simulink library "rot_grc"  (R2024a)
settings: Solver=VariableStepAuto  StartTime=0.0  StopTime=10.0  RelTol=1e-3
undefined symbols (not defined in the file or in its folder): AROT_ParkCompAngle_X_rpm, ENUM_SENSORFOCMODE_RDCALIGN, KFOC_PolePairs_p, KROT_agOffset_C, KROT_bUseVariableFc_flg, KROT_CurLoopPrd_t, KROT_RotAngleE_rad_ovrdflg, KROT_RotAngleE_rad_ovrdval, KROT_RotSpdMRaw_rpm_ovrdflg, KROT_RotSpdMRaw_rpm_ovrdval, KROT_SpdCutoffFreq_Hz, MROT_ParkCompAngle_Y_rad, MROT_VolPosnOffsWiSpd_Y_deg, ZERO_FLOAT
libraries: GRC_Lib x1
settings Model: Creator=FVT22063  LastModifiedBy=FVT22063

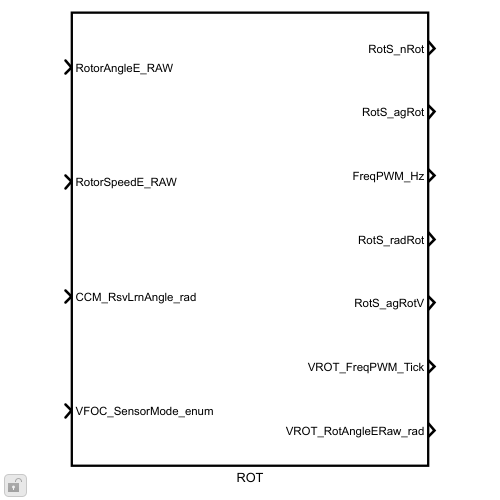
[thumbnail: Simulink's stored preview of the top-level diagram]
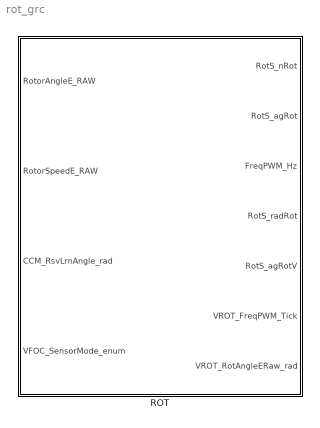
== system rot_grc ==
  ROT : Subsystem  TreatAsAtomicUnit=on

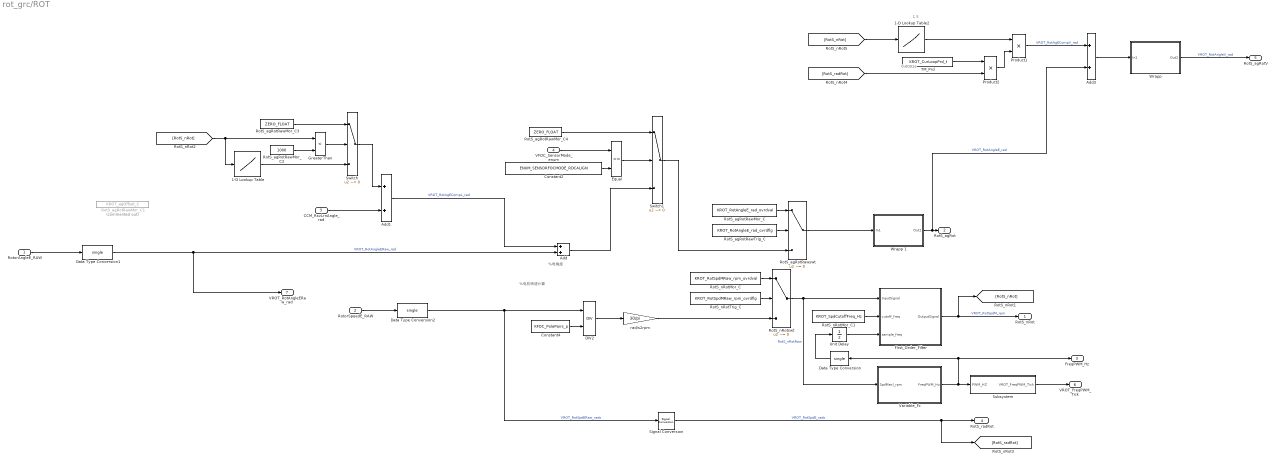
== system rot_grc/ROT ==
  note: 1.5
  note: 0.0001s
  note: %电机转速计算
  note: %电角度
  RotorAngleE_RAW : Inport
  RotorSpeedE_RAW : Inport  Port=2
  CCM_RsvLrnAngle_rad : Inport  Port=3  OutDataTypeStr=single
  VFOC_SensorMode_enum : Inport  Port=4
  1-D Lookup Table : Lookup_n-D  NumberOfTableDimensions=1  BreakpointsForDimension1=AROT_ParkCompAngle_X_rpm  Table=MROT_ParkCompAngle_Y_rad  ExtrapMethod=Clip  UseLastTableValue=on  InternalRulePriority=Speed  RndMeth=Simplest
  1-D Lookup Table2 : Lookup_n-D  NumberOfTableDimensions=1  BreakpointsForDimension1=AROT_ParkCompAngle_X_rpm  Table=MROT_VolPosnOffsWiSpd_Y_deg  ExtrapMethod=Clip  UseLastTableValue=on  InternalRulePriority=Speed  RndMeth=Simplest
  Add : Sum
  Add1 : Sum
  Add3 : Sum
  Constant2 : Constant  Value=ENUM_SENSORFOCMODE_RDCALIGN
  Constant4 : Constant  Value=KFOC_PolePairs_p
  DIV2 : GRC_Lib/ArithmeticOperations/DIV  MinDivVal=1e-15  IpDT=single
  Data Type Conversion : DataTypeConversion  OutDataTypeStr=single  SaturateOnIntegerOverflow=off  RndMeth=Floor
  Data Type Conversion1 : DataTypeConversion  OutDataTypeStr=single  SaturateOnIntegerOverflow=off  RndMeth=Floor
  Data Type Conversion2 : DataTypeConversion  OutDataTypeStr=single  SaturateOnIntegerOverflow=off  RndMeth=Floor
  Equal : RelationalOperator  Operator===  OutDataTypeStr=boolean  RndMeth=Simplest  InputSameDT=off
  First_Order_Filter : Subsystem  AncestorBlock=Library/First_Order_Filter  TreatAsAtomicUnit=on  RTWFcnName=First_Order_Filter
      settings: RTWFcnNameOpts=User specified
  GreaterThan : RelationalOperator  Operator=<  OutDataTypeStr=boolean  RndMeth=Simplest  InputSameDT=off
  Product1 : Product  RndMeth=Zero
  Product2 : Product  RndMeth=Zero
  RotS_agRotRawMor_C : Constant  Value=KROT_RotAngleE_rad_ovrdval
  RotS_agRotRawMor_C1 : Constant  Commented=on  Value=KROT_agOffset_C
  RotS_agRotRawMor_C2 : Constant  Value=1000
  RotS_agRotRawMor_C3 : Constant  Value=ZERO_FLOAT
  RotS_agRotRawMor_C4 : Constant  Value=ZERO_FLOAT
  RotS_agRotRawTrig_C : Constant  Value=KROT_RotAngleE_rad_ovrdflg
  RotS_agRotRawswt : Switch  Criteria=u2 ~= 0  SaturateOnIntegerOverflow=off  InputSameDT=off
  RotS_nRotMor_C : Constant  Value=KROT_RotSpdMRaw_rpm_ovrdval
  RotS_nRotMor_C1 : Constant  Value=KROT_SpdCutoffFreq_Hz  OutDataTypeStr=single
  RotS_nRotTrig_C : Constant  Value=KROT_RotSpdMRaw_rpm_ovrdflg
  RotS_nRotswt : Switch  Criteria=u2 ~= 0  SaturateOnIntegerOverflow=off  InputSameDT=off
  Signal Conversion : SignalConversion  OverrideOpt=off
  Subsystem : Subsystem
  Switch : Switch  Criteria=u2 ~= 0  SaturateOnIntegerOverflow=off  InputSameDT=off
  Switch1 : Switch  Criteria=u2 ~= 0  SaturateOnIntegerOverflow=off  InputSameDT=off
  TM_Prd : Constant  Value=KROT_CurLoopPrd_t  OutDataTypeStr=single
  Unit Delay : UnitDelay  InitialCondition=5000  SampleTime=-1  HasFrameUpgradeWarning=on
  Variable_Fc : Subsystem
  "Wrapp " : Subsystem
  Wrapp 1 : Subsystem
  rad/s2rpm : Gain  Gain=30/pi
  RotS_nRot : Outport  OutDataTypeStr=single  VectorParamsAs1DForOutWhenUnconnected=off
  RotS_agRot : Outport  Port=2  OutDataTypeStr=single  VectorParamsAs1DForOutWhenUnconnected=off
  FreqPWM_Hz : Outport  Port=3  OutDataTypeStr=uint16  VectorParamsAs1DForOutWhenUnconnected=off
  RotS_radRot : Outport  Port=4  OutDataTypeStr=single  VectorParamsAs1DForOutWhenUnconnected=off
  RotS_agRotV : Outport  Port=5
  VROT_FreqPWM_Tick : Outport  Port=6  VectorParamsAs1DForOutWhenUnconnected=off
  VROT_RotAngleERaw_rad : Outport  Port=7
  wires:
  RotS_nRotMor_C/1 -> RotS_nRotswt/1
  RotS_nRotTrig_C/1 -> RotS_nRotswt/2
  Constant4/1 -> DIV2/2
  DIV2/1 -> rad/s2rpm/1
  RotS_agRotRawMor_C/1 -> RotS_agRotRawswt/1
  RotS_agRotRawTrig_C/1 -> RotS_agRotRawswt/2
  rad/s2rpm/1 -> RotS_nRotswt/3
  RotorAngleE_RAW/1 -> Data Type Conversion1/1
  Variable_Fc/1(FreqPWM_Hz) -> Subsystem/1(PWM_HZ), Data Type Conversion/1, FreqPWM_Hz/1
  First_Order_Filter/1(OutputSignal) -> [RotS_nRot], RotS_nRot/1  "VROT_RotSpdM_rpm"
  Unit Delay/1 -> First_Order_Filter/3(sample_freq)
  RotS_nRotMor_C1/1 -> First_Order_Filter/2(cutoff_freq)
  RotS_nRotswt/1 -> Variable_Fc/1(SpdMecl_rpm), First_Order_Filter/1(InputSignal)  "RotS_nRotRaw"
  Data Type Conversion/1 -> Unit Delay/1
  Switch1/1 -> RotS_agRotRawswt/3
  [RotS_nRot] -> GreaterThan/1, 1-D Lookup Table/1
  1-D Lookup Table/1 -> Switch/3
  RotorSpeedE_RAW/1 -> Data Type Conversion2/1
  CCM_RsvLrnAngle_rad/1 -> Add1/2
  [RotS_nRot] -> 1-D Lookup Table2/1
  Product2/1 -> Product1/2
  1-D Lookup Table2/1 -> Product1/1
  TM_Prd/1 -> Product2/1
  Add3/1 -> "Wrapp "/1(In1)
  Product1/1 -> Add3/1  "VROT_RotAgECompV_rad"
  [RotS_radRot] -> Product2/2
  Signal Conversion/1 -> [RotS_radRot], RotS_radRot/1  "VROT_RotSpdE_rads"
  "Wrapp "/1(Out2) -> RotS_agRotV/1  "VROT_RotAngleV_rad"
  RotS_agRotRawswt/1 -> Wrapp 1/1(In1)
  Wrapp 1/1(Out2) -> Add3/2, RotS_agRot/1  "VROT_RotAngleE_rad"
  Subsystem/1(VROT_FreqPWM_Tick) -> VROT_FreqPWM_Tick/1
  Data Type Conversion1/1 -> VROT_RotAngleERaw_rad/1, Add/2  "VROT_RotAngleERaw_rad"
  Data Type Conversion2/1 -> Signal Conversion/1, DIV2/1  "VROT_RotSpdERaw_rads"
  RotS_agRotRawMor_C2/1 -> GreaterThan/2
  GreaterThan/1 -> Switch/2
  Switch/1 -> Add1/1
  RotS_agRotRawMor_C3/1 -> Switch/1
  Constant2/1 -> Equal/2
  VFOC_SensorMode_enum/1 -> Equal/1
  Equal/1 -> Switch1/2
  RotS_agRotRawMor_C4/1 -> Switch1/1
  Add1/1 -> Add/1  "VROT_RotAgECompL_rad"
  Add/1 -> Switch1/3

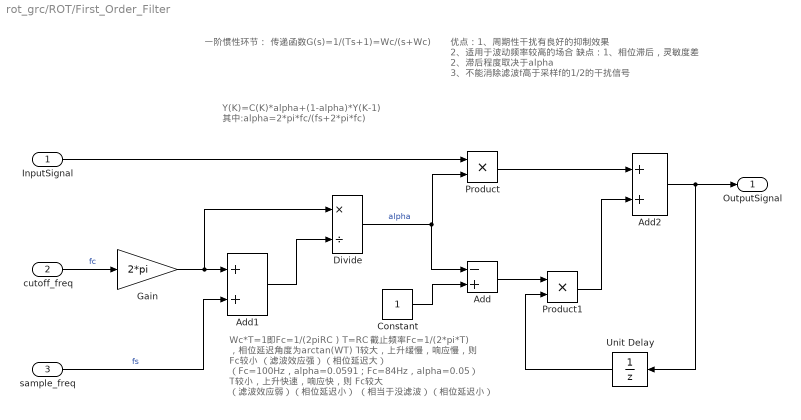
== system rot_grc/ROT/First_Order_Filter ==
  note: Y(K)=C(K)*alpha+(1-alpha)*Y(K-1)
      |
      | 其中:alpha=2*pi*fc/(fs+2*pi*fc)
  note: Wc*T=1即Fc=1/(2piRC ) T=RC
      | 截止频率Fc=1/(2*pi*T) ，相位延迟角度为arctan(WT)
      | T较大，上升缓慢，响应慢，则 Fc较小
      | （滤波效应强）（相位延迟大）
      | （Fc=100Hz，alpha=0.0591；Fc=84Hz，alpha=0.05）
      | T较小，上升快速，响应快，则 Fc较大
      | （滤波效应弱）（相位延迟小）
      | （相当于没滤波）（相位延迟小）
  note: 优点：1、周期性干扰有良好的抑制效果
      | 2、适用于波动频率较高的场合
      | 缺点：1、相位滞后，灵敏度差
      | 2、滞后程度取决于alpha
      | 3、不能消除滤波f高于采样f的1/2的干扰信号
  note: 一阶惯性环节：
      | 传递函数G(s)=1/(Ts+1)=Wc/(s+Wc)
  InputSignal : Inport  OutDataTypeStr=single
  cutoff_freq : Inport  Port=2  OutDataTypeStr=single
  sample_freq : Inport  Port=3  OutDataTypeStr=single
  Add : Sum  Inputs=-+  OutDataTypeStr=single
  Add1 : Sum  OutDataTypeStr=single
  Add2 : Sum  OutDataTypeStr=single
  Constant : Constant  OutDataTypeStr=single
  Divide : Product  Inputs=*/  OutDataTypeStr=single
  Gain : Gain  Gain=2*pi  ParamDataTypeStr=single  OutDataTypeStr=single
  Product : Product  OutDataTypeStr=single
  Product1 : Product  OutDataTypeStr=single
  Unit Delay : UnitDelay  SampleTime=-1  HasFrameUpgradeWarning=on
  OutputSignal : Outport  VectorParamsAs1DForOutWhenUnconnected=off
  wires:
  Unit Delay/1 -> Product1/2
  Add2/1 -> OutputSignal/1, Unit Delay/1
  Product/1 -> Add2/1
  Product1/1 -> Add2/2
  Add/1 -> Product1/1
  Constant/1 -> Add/2
  Divide/1 -> Product/2, Add/1  "alpha"
  Add1/1 -> Divide/2
  InputSignal/1 -> Product/1
  sample_freq/1 -> Add1/2  "fs"
  Gain/1 -> Add1/1, Divide/1
  cutoff_freq/1 -> Gain/1  "fc"

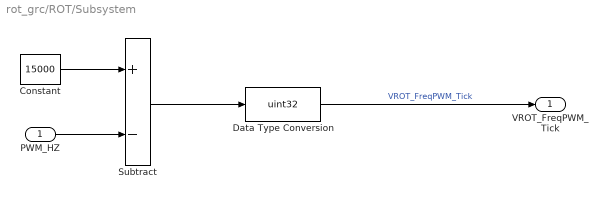
== system rot_grc/ROT/Subsystem ==
  PWM_HZ : Inport
  Constant : Constant  Value=15000
  Data Type Conversion : DataTypeConversion  OutDataTypeStr=uint32  SaturateOnIntegerOverflow=off  RndMeth=Floor
  Subtract : Sum  Inputs=+-
  VROT_FreqPWM_Tick : Outport
  wires:
  PWM_HZ/1 -> Subtract/2
  Data Type Conversion/1 -> VROT_FreqPWM_Tick/1  "VROT_FreqPWM_Tick"
  Constant/1 -> Subtract/1
  Subtract/1 -> Data Type Conversion/1

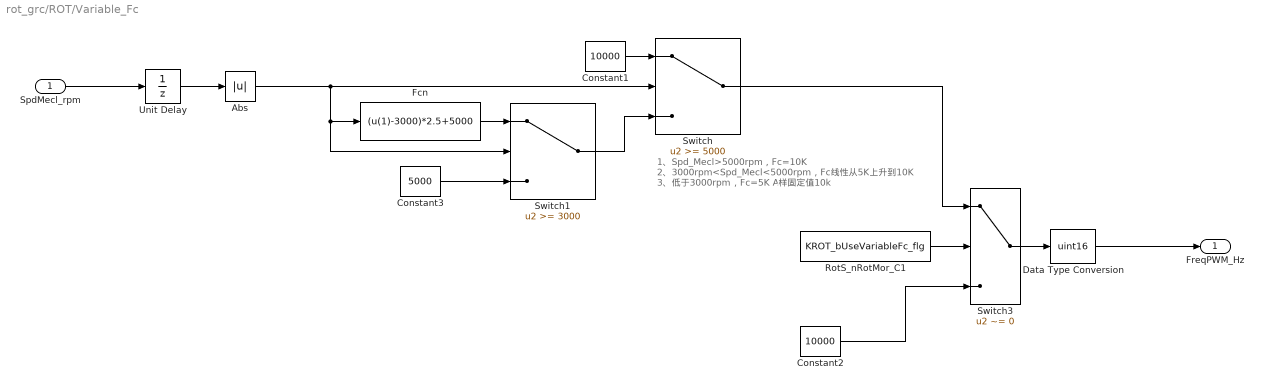
== system rot_grc/ROT/Variable_Fc ==
  note: 1、Spd_Mecl>5000rpm，Fc=10K
      | 2、3000rpm<Spd_Mecl<5000rpm，Fc线性从5K上升到10K
      | 3、低于3000rpm，Fc=5K
      | A样固定值10k
  SpdMecl_rpm : Inport  OutDataTypeStr=single
  Abs : Abs  SaturateOnIntegerOverflow=off
  Constant1 : Constant  Value=10000  OutDataTypeStr=uint16
  Constant2 : Constant  Value=10000  OutDataTypeStr=uint16
  Constant3 : Constant  Value=5000  OutDataTypeStr=uint16
  Data Type Conversion : DataTypeConversion  OutDataTypeStr=uint16  SaturateOnIntegerOverflow=off  RndMeth=Floor
  Fcn : Fcn  Expr=(u(1)-3000)*2.5+5000
  RotS_nRotMor_C1 : Constant  Value=KROT_bUseVariableFc_flg  OutDataTypeStr=single
  Switch : Switch  Threshold=5000  SaturateOnIntegerOverflow=off  InputSameDT=off
  Switch1 : Switch  Threshold=3000  SaturateOnIntegerOverflow=off  InputSameDT=off
  Switch3 : Switch  Criteria=u2 ~= 0  SaturateOnIntegerOverflow=off  InputSameDT=off
  Unit Delay : UnitDelay  SampleTime=-1  HasFrameUpgradeWarning=on
  FreqPWM_Hz : Outport  OutDataTypeStr=uint16  VectorParamsAs1DForOutWhenUnconnected=off
  wires:
  SpdMecl_rpm/1 -> Unit Delay/1
  Abs/1 -> Fcn/1, Switch1/2, Switch/2
  Constant1/1 -> Switch/1
  Switch3/1 -> Data Type Conversion/1
  Switch1/1 -> Switch/3
  Fcn/1 -> Switch1/1
  Constant3/1 -> Switch1/3
  Data Type Conversion/1 -> FreqPWM_Hz/1
  RotS_nRotMor_C1/1 -> Switch3/2
  Constant2/1 -> Switch3/3
  Switch/1 -> Switch3/1
  Unit Delay/1 -> Abs/1

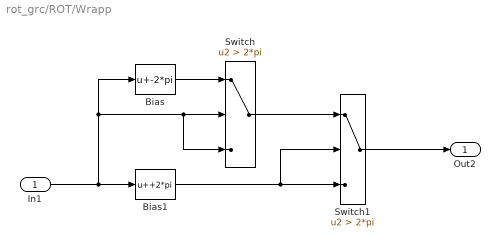
== system rot_grc/ROT/Wrapp  ==
  In1 : Inport
  Bias : Bias  Bias=-2*pi  SaturateOnIntegerOverflow=off
  Bias1 : Bias  Bias=+2*pi  SaturateOnIntegerOverflow=off
  Switch : Switch  Criteria=u2 > Threshold  Threshold=2*pi  SaturateOnIntegerOverflow=off  InputSameDT=off
  Switch1 : Switch  Criteria=u2 > Threshold  Threshold=2*pi  SaturateOnIntegerOverflow=off  InputSameDT=off
  Out2 : Outport  VectorParamsAs1DForOutWhenUnconnected=off
  wires:
  Switch/1 -> Switch1/1
  Bias/1 -> Switch/1
  In1/1 -> Bias1/1, Bias/1, Switch/3, Switch/2
  Bias1/1 -> Switch1/2, Switch1/3
  Switch1/1 -> Out2/1

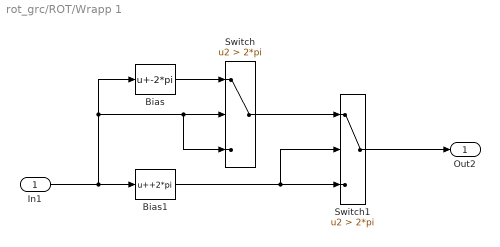
== system rot_grc/ROT/Wrapp 1 ==
  In1 : Inport
  Bias : Bias  Bias=-2*pi  SaturateOnIntegerOverflow=off
  Bias1 : Bias  Bias=+2*pi  SaturateOnIntegerOverflow=off
  Switch : Switch  Criteria=u2 > Threshold  Threshold=2*pi  SaturateOnIntegerOverflow=off  InputSameDT=off
  Switch1 : Switch  Criteria=u2 > Threshold  Threshold=2*pi  SaturateOnIntegerOverflow=off  InputSameDT=off
  Out2 : Outport  VectorParamsAs1DForOutWhenUnconnected=off
  wires:
  Switch1/1 -> Out2/1
  Bias1/1 -> Switch1/3, Switch1/2
  In1/1 -> Switch/2, Switch/3, Bias/1, Bias1/1
  Bias/1 -> Switch/1
  Switch/1 -> Switch1/1
